simulink model "Full_system"  (Simulink 8.9)
settings: Solver=FixedStepAuto  StartTime=0.0  StopTime=10.0  FixedStep=T  RelTol=1e-3
values from neighbouring files (symbols this model uses):
  A = [0 1 ; 0 -1/tau]    [get_controller.m]
  B = [0 ; km/tau]    [get_controller.m]
  C = [1 0]    [get_controller.m]
  G = G3    [get_controller.m]
  H = H3    [get_controller.m]
  T = 0.2    [full_system.mat]    (also in get_controller.m)
undefined symbols (not defined in the file or in its folder): K1, Ke, left_deadzone_m, left_deadzone_p, right_deadzone_m, right_deadzone_p
settings Model: SuppressorTable=22 serialization::archive 11 0 6 0 0 0 11 0  Creator=rafael  LastModifiedBy=rafael
settings DataIOCC: LimitDataPoints=off  SaveFormat=Dataset  SignalLoggingSaveFormat=Dataset
settings OptimizationCC: LifeSpan=auto
settings DebuggingCC: UnderspecifiedInitializationDetection=Simplified  MergeDetectMultiDrivingBlocksExec=error  MaxConsecutiveZCsMsg=none  FcnCallInpInsideContextMsg=error  StateNameClashWarn=none  SFUnexpectedBacktrackingDiag=error  SFNoUnconditionalDefaultTransitionDiag=error  SFExecutionAtInitializationDiag=warning
settings HardwareCC: ProdBitPerPointer=64  ProdBitPerSizeT=64  ProdBitPerPtrDiffT=64  ProdLargestAtomicFloat=Float  ProdIntDivRoundTo=Zero  ProdEndianess=LittleEndian  ProdWordSize=64  ProdHWDeviceType=Intel->x86-64 (Windows64)
settings ModelReferenceCC: PropagateSignalLabelsOutOfModel=on
settings GRTTargetCC: TargetLangStandard=C99 (ISO)  GeneratePreprocessorConditionals=Use local settings  CombineOutputUpdateFcns=on  GRTInterface=off
settings ConfigComp: CovMetricSettings=dwe  CovHtmlReporting=off  CovSaveCumulativeToWorkspaceVar=off  CovSaveSingleToWorkspaceVar=off  CovExternalEMLEnable=on

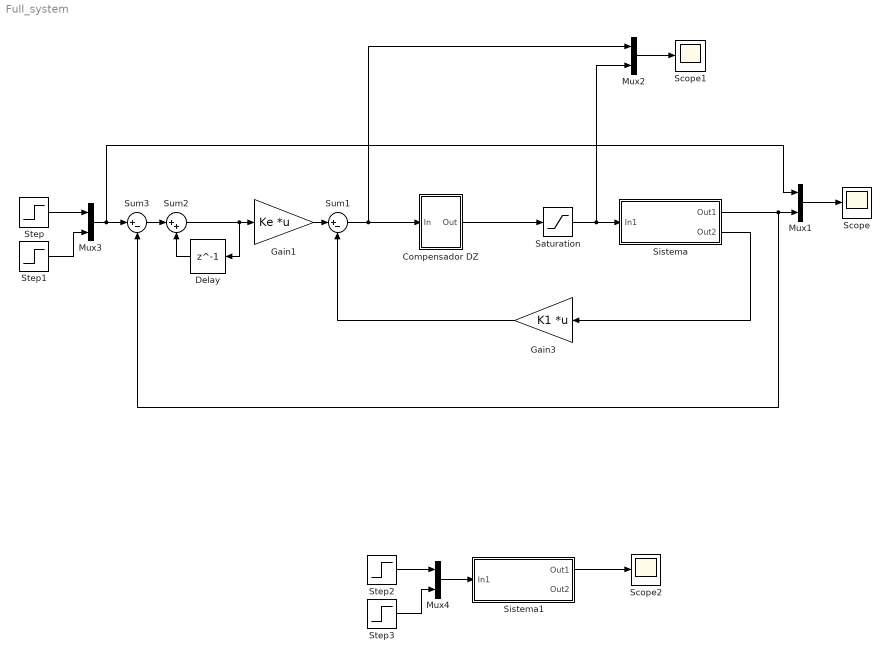
== system Full_system ==
  Compensador DZ : Subsystem
  Delay : Delay  DelayLength=1
  Gain1 : Gain  Gain=Ke  Multiplication=Matrix(K*u)
  Gain3 : Gain  Gain=K1  Multiplication=Matrix(K*u)
  Mux{1..4} (4 alike) : Mux  Inputs=2
  Saturation : Saturate  UpperLimit=7  LowerLimit=-7
  Scope : Scope
  Scope1 : Scope
  Scope2 : Scope
  Sistema : Subsystem
  Sistema1 : Subsystem
  Step : Step  After=5  SampleTime=T
  Step1 : Step  After=0  SampleTime=T
  Step2 : Step  After=5  SampleTime=T
  Step3 : Step  After=5  SampleTime=T
  Sum1 : Sum  Inputs=|+-
  Sum2 : Sum  Inputs=|++
  Sum3 : Sum  Inputs=|+-
  wires:
  Step/1 -> Mux3/1
  Step1/1 -> Mux3/2
  Mux1/1 -> Scope/1
  Gain3/1 -> Sum1/2
  Mux2/1 -> Scope1/1
  Sum1/1 -> Compensador DZ/1(In), Mux2/1
  Mux3/1 -> Sum3/1, Mux1/1
  Gain1/1 -> Sum1/1
  Compensador DZ/1(Out) -> Saturation/1
  Saturation/1 -> Mux2/2, Sistema/1(In1)
  Sum2/1 -> Delay/1, Gain1/1
  Delay/1 -> Sum2/2
  Sum3/1 -> Sum2/1
  Sistema/1(Out1) -> Sum3/2, Mux1/2
  Sistema/2(Out2) -> Gain3/1
  Step2/1 -> Mux4/1
  Step3/1 -> Mux4/2
  Mux4/1 -> Sistema1/1(In1)
  Sistema1/1(Out1) -> Scope2/1

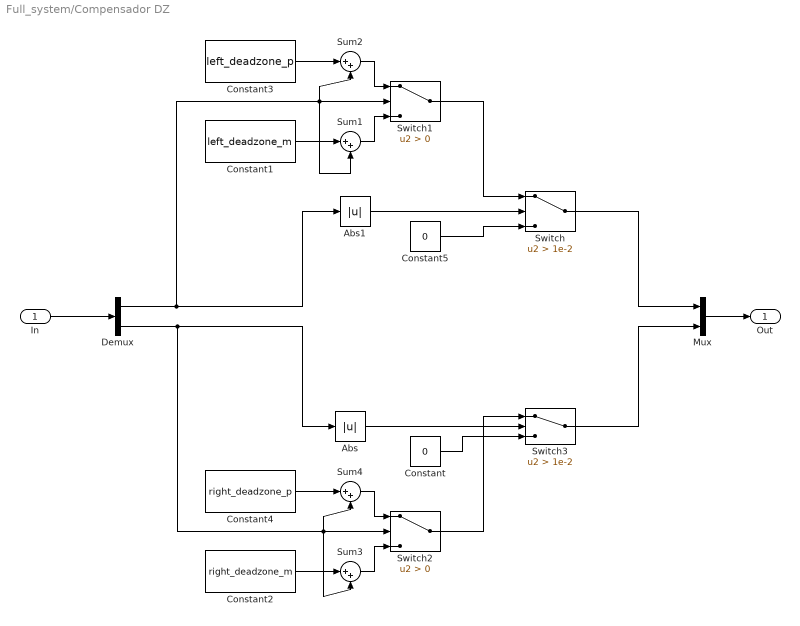
== system Full_system/Compensador DZ ==
  In : Inport
  Abs : Abs
  Abs1 : Abs
  Constant : Constant  Value=0  SampleTime=-1
  Constant1 : Constant  Value=left_deadzone_m  SampleTime=-1
  Constant2 : Constant  Value=right_deadzone_m  SampleTime=-1
  Constant3 : Constant  Value=left_deadzone_p  SampleTime=-1
  Constant4 : Constant  Value=right_deadzone_p  SampleTime=-1
  Constant5 : Constant  Value=0  SampleTime=-1
  Demux : Demux  Outputs=2
  Mux : Mux  Inputs=2
  Sum{1..4} (4 alike) : Sum  Inputs=|++
  Switch : Switch  Criteria=u2 > Threshold  Threshold=1e-2
  Switch1 : Switch  Criteria=u2 > Threshold
  Switch2 : Switch  Criteria=u2 > Threshold
  Switch3 : Switch  Criteria=u2 > Threshold  Threshold=1e-2  RndMeth=Round
  Out : Outport
  wires:
  Sum2/1 -> Switch1/1
  Constant3/1 -> Sum2/1
  Constant1/1 -> Sum1/1
  Sum1/1 -> Switch1/3
  Switch1/1 -> Switch/1
  Switch2/1 -> Switch3/1
  Constant2/1 -> Sum3/1
  Sum3/1 -> Switch2/3
  Constant4/1 -> Sum4/1
  Sum4/1 -> Switch2/1
  Switch/1 -> Mux/1
  Switch3/1 -> Mux/2
  Mux/1 -> Out/1
  In/1 -> Demux/1
  Demux/2 -> Abs/1, Sum3/2, Sum4/2, Switch2/2
  Constant/1 -> Switch3/3
  Abs/1 -> Switch3/2
  Abs1/1 -> Switch/2
  Constant5/1 -> Switch/3
  Demux/1 -> Switch1/2, Sum2/2, Sum1/2, Abs1/1

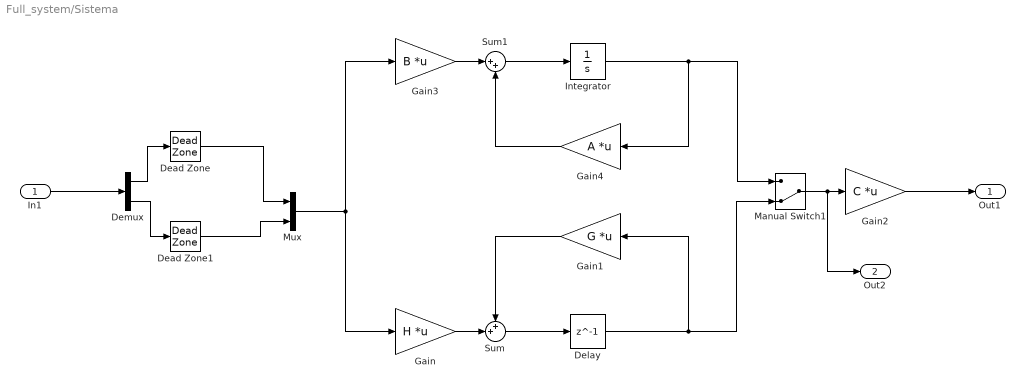
== system Full_system/Sistema ==
  In1 : Inport
  Dead Zone : DeadZone  LowerValue=left_deadzone_m  UpperValue=left_deadzone_p  SaturateOnIntegerOverflow=on
  Dead Zone1 : DeadZone  LowerValue=right_deadzone_m  UpperValue=right_deadzone_p  SaturateOnIntegerOverflow=on
  Delay : Delay  DelayLength=1
  Demux : Demux  Outputs=2
  Gain : Gain  Gain=H  Multiplication=Matrix(K*u)
  Gain1 : Gain  Gain=G  Multiplication=Matrix(K*u)
  Gain2 : Gain  Gain=C  Multiplication=Matrix(K*u)
  Gain3 : Gain  Gain=B  Multiplication=Matrix(K*u)
  Gain4 : Gain  Gain=A  Multiplication=Matrix(K*u)
  Integrator : Integrator
  Manual Switch1 : ManualSwitch  CurrentSetting=0
  Mux : Mux  Inputs=2
  Sum : Sum  Inputs=++|
  Sum1 : Sum  Inputs=|++
  Out1 : Outport
  Out2 : Outport  Port=2
  wires:
  Delay/1 -> Manual Switch1/2, Gain1/1
  Sum/1 -> Delay/1
  Gain2/1 -> Out1/1
  Demux/1 -> Dead Zone/1
  Demux/2 -> Dead Zone1/1
  Dead Zone/1 -> Mux/1
  Dead Zone1/1 -> Mux/2
  Gain4/1 -> Sum1/2
  Gain3/1 -> Sum1/1
  Integrator/1 -> Gain4/1, Manual Switch1/1
  Sum1/1 -> Integrator/1
  Manual Switch1/1 -> Out2/1, Gain2/1
  Gain/1 -> Sum/2
  Gain1/1 -> Sum/1
  Mux/1 -> Gain/1, Gain3/1
  In1/1 -> Demux/1

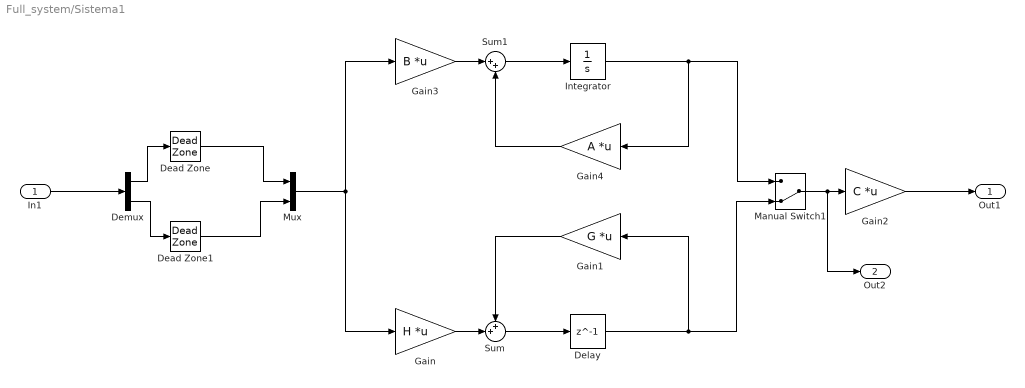
== system Full_system/Sistema1 ==
  In1 : Inport
  Dead Zone : DeadZone  LowerValue=left_deadzone_m  UpperValue=left_deadzone_p  SaturateOnIntegerOverflow=on
  Dead Zone1 : DeadZone  LowerValue=right_deadzone_m  UpperValue=right_deadzone_p  SaturateOnIntegerOverflow=on
  Delay : Delay  DelayLength=1
  Demux : Demux  Outputs=2
  Gain : Gain  Gain=H  Multiplication=Matrix(K*u)
  Gain1 : Gain  Gain=G  Multiplication=Matrix(K*u)
  Gain2 : Gain  Gain=C  Multiplication=Matrix(K*u)
  Gain3 : Gain  Gain=B  Multiplication=Matrix(K*u)
  Gain4 : Gain  Gain=A  Multiplication=Matrix(K*u)
  Integrator : Integrator
  Manual Switch1 : ManualSwitch  CurrentSetting=0
  Mux : Mux  Inputs=2
  Sum : Sum  Inputs=++|
  Sum1 : Sum  Inputs=|++
  Out1 : Outport
  Out2 : Outport  Port=2
  wires:
  Delay/1 -> Manual Switch1/2, Gain1/1
  Sum/1 -> Delay/1
  Gain2/1 -> Out1/1
  Demux/1 -> Dead Zone/1
  Demux/2 -> Dead Zone1/1
  Dead Zone/1 -> Mux/1
  Dead Zone1/1 -> Mux/2
  Gain4/1 -> Sum1/2
  Gain3/1 -> Sum1/1
  Integrator/1 -> Gain4/1, Manual Switch1/1
  Sum1/1 -> Integrator/1
  Manual Switch1/1 -> Out2/1, Gain2/1
  Gain/1 -> Sum/2
  Gain1/1 -> Sum/1
  Mux/1 -> Gain/1, Gain3/1
  In1/1 -> Demux/1
